simulink model "fifo3"  (R2023a)
settings: Solver=VariableStepAuto  StartTime=0.0  StopTime=10.0  RelTol=1e-3
libraries: NSA_DEVS_SINKS_ATOMIC x6, NSA_DEVS_ROUTING_ATOMIC x3, NSA_DEVS_LOGISTICS_COUPLED x3, NSA_DEVS_SOURCES_ATOMIC x1, NSA_DEVS_LOGISTICS_ATOMIC x1
settings Model: Creator=david  LastModifiedBy=david
settings OptimizationCC: ReuseModelBlockBuffer=off

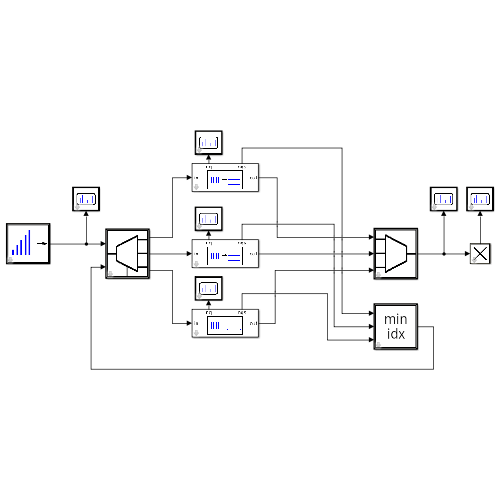
[thumbnail: Simulink's stored preview of the top-level diagram]
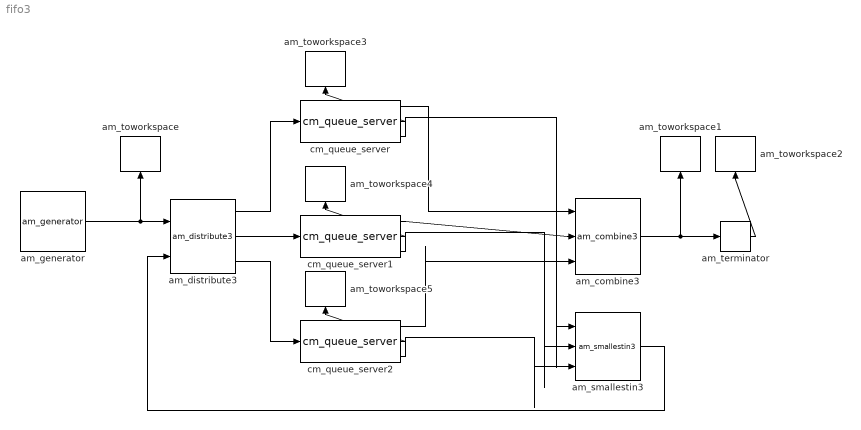
== system fifo3 ==
  am_combine3 : NSA_DEVS_ROUTING_ATOMIC/am_combine3  tD=[0,1]  tau=[0,1]  debug=0
      settings: SourceProductName=NSA_DEVS
  am_distribute3 : NSA_DEVS_ROUTING_ATOMIC/am_distribute3  port0=1  tau=[0,1]  debug=0
      settings: SourceProductName=NSA_DEVS
  am_generator : NSA_DEVS_SOURCES_ATOMIC/am_generator  tG=1  n0=1  nG=13  tau=[0,1]  debug=0
      settings: SourceProductName=NSA_DEVS
  am_smallestin3 : NSA_DEVS_ROUTING_ATOMIC/am_smallestin3  val0=0  tau=[0,1]  debug=0
      settings: SourceProductName=NSA_DEVS
  am_terminator : NSA_DEVS_LOGISTICS_ATOMIC/am_terminator  tau=[0,1]  debug=0
      settings: SourceProductName=NSA_DEVS
  am_toworkspace : NSA_DEVS_SINKS_ATOMIC/am_toworkspace  varname="\"gen_out\""  t0=0  format="\"vector\""  tau=[0,5]  debug=0
      settings: SourceProductName=NSA_DEVS
  am_toworkspace1 : NSA_DEVS_SINKS_ATOMIC/am_toworkspace  varname="\"output\""  t0=0  format="\"vector\""  tau=[0,5]  debug=0
      settings: SourceProductName=NSA_DEVS
  am_toworkspace2 : NSA_DEVS_SINKS_ATOMIC/am_toworkspace  varname="\"thrput\""  t0=0  format="\"vector\""  tau=[0,5]  debug=0
      settings: SourceProductName=NSA_DEVS
  am_toworkspace3 : NSA_DEVS_SINKS_ATOMIC/am_toworkspace  varname="\"nq1\""  t0=0  format="\"vector\""  tau=[0,5]  debug=0
      settings: SourceProductName=NSA_DEVS
  am_toworkspace4 : NSA_DEVS_SINKS_ATOMIC/am_toworkspace  varname="\"nq2\""  t0=0  format="\"vector\""  tau=[0,5]  debug=0
      settings: SourceProductName=NSA_DEVS
  am_toworkspace5 : NSA_DEVS_SINKS_ATOMIC/am_toworkspace  varname="\"nq3\""  t0=0  format="\"vector\""  tau=[0,5]  debug=0
      settings: SourceProductName=NSA_DEVS
  cm_queue_server : NSA_DEVS_LOGISTICS_COUPLED/cm_queue_server  ts=4.5  tau=[0,1]  debug=0
      settings: SourceProductName=NSA_DEVS
  cm_queue_server1 : NSA_DEVS_LOGISTICS_COUPLED/cm_queue_server  ts=4.5  tau=[0,1]  debug=0
      settings: SourceProductName=NSA_DEVS
  cm_queue_server2 : NSA_DEVS_LOGISTICS_COUPLED/cm_queue_server  ts=4.5  tau=[0,1]  debug=0
      settings: SourceProductName=NSA_DEVS
  wires:
  am_distribute3/1 -> cm_queue_server/1
  am_distribute3/2 -> cm_queue_server1/1
  am_distribute3/3 -> cm_queue_server2/1
  cm_queue_server1/1 -> am_combine3/2
  cm_queue_server/1 -> am_combine3/1
  cm_queue_server2/1 -> am_combine3/3
  cm_queue_server/3 -> am_smallestin3/1
  cm_queue_server1/3 -> am_smallestin3/2
  cm_queue_server2/3 -> am_smallestin3/3
  am_smallestin3/1 -> am_distribute3/2
  am_generator/1 -> am_toworkspace/1, am_distribute3/1
  am_combine3/1 -> am_toworkspace1/1, am_terminator/1
  am_terminator/1 -> am_toworkspace2/1
  cm_queue_server/2 -> am_toworkspace3/1
  cm_queue_server1/2 -> am_toworkspace4/1
  cm_queue_server2/2 -> am_toworkspace5/1
